simulink model "six_plus_six_AcmsteeringV10_main"  (R2014a)
settings: Solver=FixedStepDiscrete  StartTime=0.0  StopTime=10.0  FixedStep=0.0005  RelTol=1e-3
InitFcn:
  | Veh_Par_wxt
values from neighbouring files (symbols this model uses):
  acc_spdctl = [0 100]    [Veh_Par_wxt.m]
  ag_thr = ecucoder_cal(ag_thr)    [Veh_Par_wxt.m]
  B = 1.8    [Veh_Par_wxt.m]
  bra_em = 100    [Veh_Par_wxt.m]
  bra_pre_gz2 = 100/3    (= 33.3333333333)    [Veh_Par_wxt.m]
  bra_pre_gz34 = 10/3    (= 3.33333333333)    [Veh_Par_wxt.m]
  bra_pre_yd = 10/2    (= 5)    [Veh_Par_wxt.m]
  brakepre_dem_data = [0 1 2 3 4 5 6 7 8 9 10]    [Veh_Par_wxt.m]
  brakeTrq_dem_data = [0 125 251 376 502 627 753 878 1004 1129 1255]    [Veh_Par_wxt.m]
  bratrq_max = 4*1255    (= 5020)    [Veh_Par_wxt.m]
  eff_tran = 0.9    [Veh_Par_wxt.m]
  ESP_switch = ecucoder_cal(ESP_switch)    [Veh_Par_wxt.m]
  G = Mass*g    (= 15696)    [Veh_Par_wxt.m]
  kd1 = ecucoder_cal(kd1)    [Veh_Par_wxt.m]
  kd2 = 0    [Veh_Par_wxt.m]
  ki1 = ecucoder_cal(ki1)    [Veh_Par_wxt.m]
  ki2 = 1    [Veh_Par_wxt.m]
  kp1 = ecucoder_cal(kp1)    [Veh_Par_wxt.m]
  kp2 = 300    [Veh_Par_wxt.m]
  L = L1+L2    (= 2.9)    [Veh_Par_wxt.m]
  premax = 100    [Veh_Par_wxt.m]
  Radius = 0.4572/2    (= 0.2286)    [Veh_Par_wxt.m]
  RC_switch = ecucoder_cal(RC_switch)    [Veh_Par_wxt.m]
  s_opt_yi = 0.15    [Veh_Par_wxt.m]
  s_opt_zhuan = 0.8    [Veh_Par_wxt.m]
  s_opt_zhuan_add = 0.05    [Veh_Par_wxt.m]
  s_opt_zhuan_table = [0.8 0.8 0.3 0.3]    [Veh_Par_wxt.m]
  spd_map_mot = [0 499.85 999.79 1500 2000 2500 3000 3500 4000 4500 4999.8 5999.8]    [Veh_Par_wxt.m]
  spd_spdctl = [0 500]    [Veh_Par_wxt.m]
  speed_thr_park = 5/3.6/Radius*tras_ratio*30/pi    (= 464.143899364)    [Veh_Par_wxt.m]
  TCS_switch = ecucoder_cal(TCS_switch)    [Veh_Par_wxt.m]
  tras_ratio = 8    [Veh_Par_wxt.m]
  trq_map_mot = [70.5 70.012 71.154 65.797 53.917 45.159 38.073 32.685 27.48 17.133 14.949 10.07]    [Veh_Par_wxt.m]
  trqmax_yd = 70.5    [Veh_Par_wxt.m]
  trqmax_zx = 70.5    [Veh_Par_wxt.m]
  trqmaxneg = -70.5    [Veh_Par_wxt.m]
  v_gain = 0.9    [Veh_Par_wxt.m]
  v_table = [0 5 20 100]    [Veh_Par_wxt.m]
  v_thr_park = 5    [Veh_Par_wxt.m]
  zhidong_bianmazhi = [-140000 750000]    [Veh_Par_wxt.m]
  zhidong_down = -140000    [Veh_Par_wxt.m]
  zhidong_up = 750000    [Veh_Par_wxt.m]
  zhidong_youmen = [0 100]    [Veh_Par_wxt.m]
  zhuanxiang_bianmazhi = [-400000 0 400000]    [Veh_Par_wxt.m]
  zhuanxiang_down = -400000    [Veh_Par_wxt.m]
  zhuanxiang_up = 400000    [Veh_Par_wxt.m]
  zhuanxiang_youmen = [-100 0 100]    [Veh_Par_wxt.m]
undefined symbols (not defined in the file or in its folder): ecucoder_acal, guzhang_lf, guzhang_lm, guzhang_lr, guzhang_rf, guzhang_rm, guzhang_rr, myFIS
libraries: simulink x979, ec5744lib x59, fuzblock x2
(part 13 of 27)

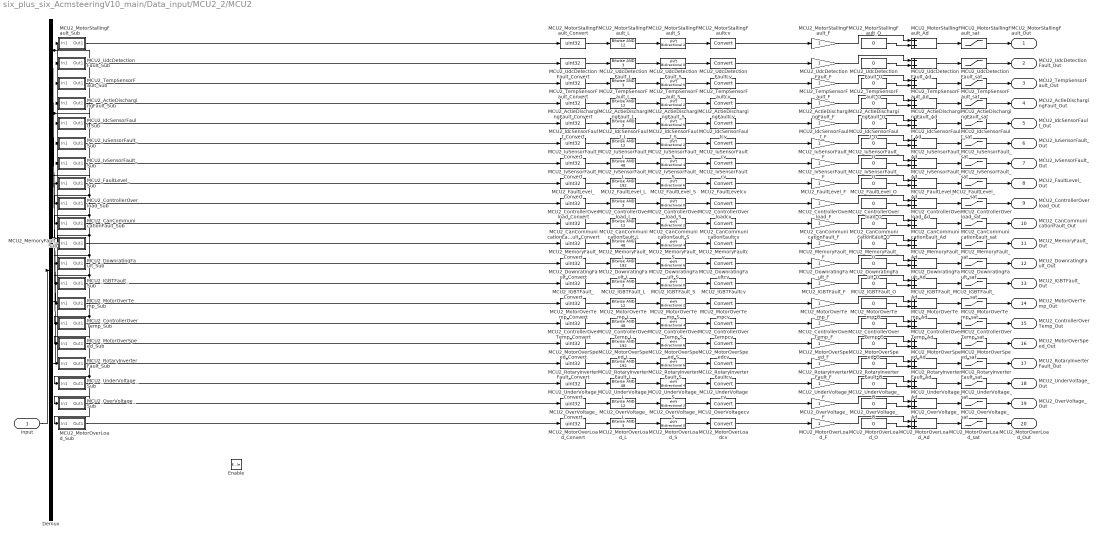
== system six_plus_six_AcmsteeringV10_main/Data_input/MCU2_2/MCU2 ==
  input : Inport
  Enable : EnablePort
  Demux : Demux  Outputs=8
  MCU2_ActieDischargingFault_Ad : Sum
  MCU2_ActieDischargingFault_Convert : DataTypeConversion  OutDataTypeStr=uint32
  MCU2_ActieDischargingFault_F : Gain
  MCU2_ActieDischargingFault_L : simulink/Logic and Bit Operations/Bitwise Operator  logicop=AND  UseBitMask=on  BitMask=12  BitMaskRealWorld=Stored Integer
  MCU2_ActieDischargingFault_O : Constant  Value=0  OutDataTypeStr=single
  MCU2_ActieDischargingFault_S : ArithShift  BitShiftNumber=2
  MCU2_ActieDischargingFault_Sub : Subsystem
  MCU2_ActieDischargingFault_sat : Saturate  UpperLimit=3  LowerLimit=0
  MCU2_ActieDischargingFaultcv : DataTypeConversion
  MCU2_CanCommunicationFault_Ad : Sum
  MCU2_CanCommunicationFault_Convert : DataTypeConversion  OutDataTypeStr=uint32
  MCU2_CanCommunicationFault_F : Gain
  MCU2_CanCommunicationFault_L : simulink/Logic and Bit Operations/Bitwise Operator  logicop=AND  UseBitMask=on  BitMask=12  BitMaskRealWorld=Stored Integer
  MCU2_CanCommunicationFault_O : Constant  Value=0  OutDataTypeStr=single
  MCU2_CanCommunicationFault_S : ArithShift  BitShiftNumber=2
  MCU2_CanCommunicationFault_Sub : Subsystem
  MCU2_CanCommunicationFault_sat : Saturate  UpperLimit=3  LowerLimit=0
  MCU2_CanCommunicationFaultcv : DataTypeConversion
  MCU2_ControllerOverTemp_Ad : Sum
  MCU2_ControllerOverTemp_Convert : DataTypeConversion  OutDataTypeStr=uint32
  MCU2_ControllerOverTemp_F : Gain
  MCU2_ControllerOverTemp_L : simulink/Logic and Bit Operations/Bitwise Operator  logicop=AND  UseBitMask=on  BitMask=48  BitMaskRealWorld=Stored Integer
  MCU2_ControllerOverTemp_O : Constant  Value=0  OutDataTypeStr=single
  MCU2_ControllerOverTemp_S : ArithShift  BitShiftNumber=4
  MCU2_ControllerOverTemp_Sub : Subsystem
  MCU2_ControllerOverTemp_sat : Saturate  UpperLimit=3  LowerLimit=0
  MCU2_ControllerOverTempcv : DataTypeConversion
  MCU2_ControllerOverload_Ad : Sum
  MCU2_ControllerOverload_Convert : DataTypeConversion  OutDataTypeStr=uint32
  MCU2_ControllerOverload_F : Gain
  MCU2_ControllerOverload_L : simulink/Logic and Bit Operations/Bitwise Operator  logicop=AND  UseBitMask=on  BitMask=3  BitMaskRealWorld=Stored Integer
  MCU2_ControllerOverload_O : Constant  Value=0  OutDataTypeStr=single
  MCU2_ControllerOverload_S : ArithShift
  MCU2_ControllerOverload_Sub : Subsystem
  MCU2_ControllerOverload_sat : Saturate  UpperLimit=3  LowerLimit=0
  MCU2_ControllerOverloadcv : DataTypeConversion
  MCU2_DownratingFault_Ad : Sum
  MCU2_DownratingFault_Convert : DataTypeConversion  OutDataTypeStr=uint32
  MCU2_DownratingFault_F : Gain
  MCU2_DownratingFault_L : simulink/Logic and Bit Operations/Bitwise Operator  logicop=AND  UseBitMask=on  BitMask=192  BitMaskRealWorld=Stored Integer
  MCU2_DownratingFault_O : Constant  Value=0  OutDataTypeStr=single
  MCU2_DownratingFault_S : ArithShift  BitShiftNumber=6
  MCU2_DownratingFault_Sub : Subsystem
  MCU2_DownratingFault_sat : Saturate  UpperLimit=3  LowerLimit=0
  MCU2_DownratingFaultcv : DataTypeConversion
  MCU2_FaultLevel_Ad : Sum
  MCU2_FaultLevel_Convert : DataTypeConversion  OutDataTypeStr=uint32
  MCU2_FaultLevel_F : Gain
  MCU2_FaultLevel_L : simulink/Logic and Bit Operations/Bitwise Operator  logicop=AND  UseBitMask=on  BitMask=192  BitMaskRealWorld=Stored Integer
  MCU2_FaultLevel_O : Constant  Value=0  OutDataTypeStr=single
  MCU2_FaultLevel_S : ArithShift  BitShiftNumber=6
  MCU2_FaultLevel_Sub : Subsystem
  MCU2_FaultLevel_sat : Saturate  UpperLimit=3  LowerLimit=0
  MCU2_FaultLevelcv : DataTypeConversion
  MCU2_IGBTFault_Ad : Sum
  MCU2_IGBTFault_Convert : DataTypeConversion  OutDataTypeStr=uint32
  MCU2_IGBTFault_F : Gain
  MCU2_IGBTFault_L : simulink/Logic and Bit Operations/Bitwise Operator  logicop=AND  UseBitMask=on  BitMask=3  BitMaskRealWorld=Stored Integer
  MCU2_IGBTFault_O : Constant  Value=0  OutDataTypeStr=single
  MCU2_IGBTFault_S : ArithShift
  MCU2_IGBTFault_Sub : Subsystem
  MCU2_IGBTFault_sat : Saturate  UpperLimit=3  LowerLimit=0
  MCU2_IGBTFaultcv : DataTypeConversion
  MCU2_IdcSensorFault_Ad : Sum
  MCU2_IdcSensorFault_Convert : DataTypeConversion  OutDataTypeStr=uint32
  MCU2_IdcSensorFault_F : Gain
  MCU2_IdcSensorFault_L : simulink/Logic and Bit Operations/Bitwise Operator  logicop=AND  UseBitMask=on  BitMask=3  BitMaskRealWorld=Stored Integer
  MCU2_IdcSensorFault_O : Constant  Value=0  OutDataTypeStr=single
  MCU2_IdcSensorFault_S : ArithShift
  MCU2_IdcSensorFault_Sub : Subsystem
  MCU2_IdcSensorFault_sat : Saturate  UpperLimit=3  LowerLimit=0
  MCU2_IdcSensorFaultcv : DataTypeConversion
  MCU2_IuSensorFault_Ad : Sum
  MCU2_IuSensorFault_Convert : DataTypeConversion  OutDataTypeStr=uint32
  MCU2_IuSensorFault_F : Gain
  MCU2_IuSensorFault_L : simulink/Logic and Bit Operations/Bitwise Operator  logicop=AND  UseBitMask=on  BitMask=12  BitMaskRealWorld=Stored Integer
  MCU2_IuSensorFault_O : Constant  Value=0  OutDataTypeStr=single
  MCU2_IuSensorFault_S : ArithShift  BitShiftNumber=2
  MCU2_IuSensorFault_Sub : Subsystem
  MCU2_IuSensorFault_sat : Saturate  UpperLimit=3  LowerLimit=0
  MCU2_IuSensorFaultcv : DataTypeConversion
  MCU2_IvSensorFault_Ad : Sum
  MCU2_IvSensorFault_Convert : DataTypeConversion  OutDataTypeStr=uint32
  MCU2_IvSensorFault_F : Gain
  MCU2_IvSensorFault_L : simulink/Logic and Bit Operations/Bitwise Operator  logicop=AND  UseBitMask=on  BitMask=48  BitMaskRealWorld=Stored Integer
  MCU2_IvSensorFault_O : Constant  Value=0  OutDataTypeStr=single
  MCU2_IvSensorFault_S : ArithShift  BitShiftNumber=4
  MCU2_IvSensorFault_Sub : Subsystem
  MCU2_IvSensorFault_sat : Saturate  UpperLimit=3  LowerLimit=0
  MCU2_IvSensorFaultcv : DataTypeConversion
  MCU2_MemoryFault_Ad : Sum
  MCU2_MemoryFault_Convert : DataTypeConversion  OutDataTypeStr=uint32
  MCU2_MemoryFault_F : Gain
  MCU2_MemoryFault_L : simulink/Logic and Bit Operations/Bitwise Operator  logicop=AND  UseBitMask=on  BitMask=48  BitMaskRealWorld=Stored Integer
  MCU2_MemoryFault_O : Constant  Value=0  OutDataTypeStr=single
  MCU2_MemoryFault_S : ArithShift  BitShiftNumber=4
  MCU2_MemoryFault_Sub : Subsystem
  MCU2_MemoryFault_sat : Saturate  UpperLimit=3  LowerLimit=0
  MCU2_MemoryFaultcv : DataTypeConversion
  MCU2_MotorOverLoad_Ad : Sum
  MCU2_MotorOverLoad_Convert : DataTypeConversion  OutDataTypeStr=uint32
  MCU2_MotorOverLoad_F : Gain
  MCU2_MotorOverLoad_L : simulink/Logic and Bit Operations/Bitwise Operator  logicop=AND  UseBitMask=on  BitMask=3  BitMaskRealWorld=Stored Integer
  MCU2_MotorOverLoad_O : Constant  Value=0  OutDataTypeStr=single
  MCU2_MotorOverLoad_S : ArithShift
  MCU2_MotorOverLoad_Sub : Subsystem
  MCU2_MotorOverLoad_sat : Saturate  UpperLimit=3  LowerLimit=0
  MCU2_MotorOverLoadcv : DataTypeConversion
  MCU2_MotorOverSpeed_Ad : Sum
  MCU2_MotorOverSpeed_Convert : DataTypeConversion  OutDataTypeStr=uint32
  MCU2_MotorOverSpeed_F : Gain
  MCU2_MotorOverSpeed_L : simulink/Logic and Bit Operations/Bitwise Operator  logicop=AND  UseBitMask=on  BitMask=192  BitMaskRealWorld=Stored Integer
  MCU2_MotorOverSpeed_O : Constant  Value=0  OutDataTypeStr=single
  MCU2_MotorOverSpeed_S : ArithShift  BitShiftNumber=6
  MCU2_MotorOverSpeed_Sub : Subsystem
  MCU2_MotorOverSpeed_sat : Saturate  UpperLimit=3  LowerLimit=0
  MCU2_MotorOverSpeedcv : DataTypeConversion
  MCU2_MotorOverTemp_Ad : Sum
  MCU2_MotorOverTemp_Convert : DataTypeConversion  OutDataTypeStr=uint32
  MCU2_MotorOverTemp_F : Gain
  MCU2_MotorOverTemp_L : simulink/Logic and Bit Operations/Bitwise Operator  logicop=AND  UseBitMask=on  BitMask=12  BitMaskRealWorld=Stored Integer
  MCU2_MotorOverTemp_O : Constant  Value=0  OutDataTypeStr=single
  MCU2_MotorOverTemp_S : ArithShift  BitShiftNumber=2
  MCU2_MotorOverTemp_Sub : Subsystem
  MCU2_MotorOverTemp_sat : Saturate  UpperLimit=3  LowerLimit=0
  MCU2_MotorOverTempcv : DataTypeConversion
  MCU2_MotorStallingFault_Ad : Sum
  MCU2_MotorStallingFault_Convert : DataTypeConversion  OutDataTypeStr=uint32
  MCU2_MotorStallingFault_F : Gain
  MCU2_MotorStallingFault_L : simulink/Logic and Bit Operations/Bitwise Operator  logicop=AND  UseBitMask=on  BitMask=12  BitMaskRealWorld=Stored Integer
  MCU2_MotorStallingFault_O : Constant  Value=0  OutDataTypeStr=single
  MCU2_MotorStallingFault_S : ArithShift  BitShiftNumber=2
  MCU2_MotorStallingFault_Sub : Subsystem
  MCU2_MotorStallingFault_sat : Saturate  UpperLimit=3  LowerLimit=0
  MCU2_MotorStallingFaultcv : DataTypeConversion
  MCU2_OverVoltage_Ad : Sum
  MCU2_OverVoltage_Convert : DataTypeConversion  OutDataTypeStr=uint32
  MCU2_OverVoltage_F : Gain
  MCU2_OverVoltage_L : simulink/Logic and Bit Operations/Bitwise Operator  logicop=AND  UseBitMask=on  BitMask=12  BitMaskRealWorld=Stored Integer
  MCU2_OverVoltage_O : Constant  Value=0  OutDataTypeStr=single
  MCU2_OverVoltage_S : ArithShift  BitShiftNumber=2
  MCU2_OverVoltage_Sub : Subsystem
  MCU2_OverVoltage_sat : Saturate  UpperLimit=3  LowerLimit=0
  MCU2_OverVoltagecv : DataTypeConversion
  MCU2_RotaryInverterFault_Ad : Sum
  MCU2_RotaryInverterFault_Convert : DataTypeConversion  OutDataTypeStr=uint32
  MCU2_RotaryInverterFault_F : Gain
  MCU2_RotaryInverterFault_L : simulink/Logic and Bit Operations/Bitwise Operator  logicop=AND  UseBitMask=on  BitMask=192  BitMaskRealWorld=Stored Integer
  MCU2_RotaryInverterFault_O : Constant  Value=0  OutDataTypeStr=single
  MCU2_RotaryInverterFault_S : ArithShift  BitShiftNumber=6
  MCU2_RotaryInverterFault_Sub : Subsystem
  MCU2_RotaryInverterFault_sat : Saturate  UpperLimit=3  LowerLimit=0
  MCU2_RotaryInverterFaultcv : DataTypeConversion
  MCU2_TempSensorFault_Ad : Sum
  MCU2_TempSensorFault_Convert : DataTypeConversion  OutDataTypeStr=uint32
  MCU2_TempSensorFault_F : Gain
  MCU2_TempSensorFault_L : simulink/Logic and Bit Operations/Bitwise Operator  logicop=AND  UseBitMask=on  BitMask=3  BitMaskRealWorld=Stored Integer
  MCU2_TempSensorFault_O : Constant  Value=0  OutDataTypeStr=single
  MCU2_TempSensorFault_S : ArithShift
  MCU2_TempSensorFault_Sub : Subsystem
  MCU2_TempSensorFault_sat : Saturate  UpperLimit=3  LowerLimit=0
  MCU2_TempSensorFaultcv : DataTypeConversion
  MCU2_UdcDetectionFault_Ad : Sum
  MCU2_UdcDetectionFault_Convert : DataTypeConversion  OutDataTypeStr=uint32
  MCU2_UdcDetectionFault_F : Gain
  MCU2_UdcDetectionFault_L : simulink/Logic and Bit Operations/Bitwise Operator  logicop=AND  UseBitMask=on  BitMask=3  BitMaskRealWorld=Stored Integer
  MCU2_UdcDetectionFault_O : Constant  Value=0  OutDataTypeStr=single
  MCU2_UdcDetectionFault_S : ArithShift
  MCU2_UdcDetectionFault_Sub : Subsystem
  MCU2_UdcDetectionFault_sat : Saturate  UpperLimit=3  LowerLimit=0
  MCU2_UdcDetectionFaultcv : DataTypeConversion
  MCU2_UnderVoltage_Ad : Sum
  MCU2_UnderVoltage_Convert : DataTypeConversion  OutDataTypeStr=uint32
  MCU2_UnderVoltage_F : Gain
  MCU2_UnderVoltage_L : simulink/Logic and Bit Operations/Bitwise Operator  logicop=AND  UseBitMask=on  BitMask=48  BitMaskRealWorld=Stored Integer
  MCU2_UnderVoltage_O : Constant  Value=0  OutDataTypeStr=single
  MCU2_UnderVoltage_S : ArithShift  BitShiftNumber=4
  MCU2_UnderVoltage_Sub : Subsystem
  MCU2_UnderVoltage_sat : Saturate  UpperLimit=3  LowerLimit=0
  MCU2_UnderVoltagecv : DataTypeConversion
  MCU2_MotorStallingFault_Out : Outport
  MCU2_UdcDetectionFault_Out : Outport  Port=2
  MCU2_TempSensorFault_Out : Outport  Port=3
  MCU2_ActieDischargingFault_Out : Outport  Port=4
  MCU2_IdcSensorFault_Out : Outport  Port=5
  MCU2_IuSensorFault_Out : Outport  Port=6
  MCU2_IvSensorFault_Out : Outport  Port=7
  MCU2_FaultLevel_Out : Outport  Port=8
  MCU2_ControllerOverload_Out : Outport  Port=9
  MCU2_CanCommunicationFault_Out : Outport  Port=10
  MCU2_MemoryFault_Out : Outport  Port=11
  MCU2_DownratingFault_Out : Outport  Port=12
  MCU2_IGBTFault_Out : Outport  Port=13
  MCU2_MotorOverTemp_Out : Outport  Port=14
  MCU2_ControllerOverTemp_Out : Outport  Port=15
  MCU2_MotorOverSpeed_Out : Outport  Port=16
  MCU2_RotaryInverterFault_Out : Outport  Port=17
  MCU2_UnderVoltage_Out : Outport  Port=18
  MCU2_OverVoltage_Out : Outport  Port=19
  MCU2_MotorOverLoad_Out : Outport  Port=20
  wires:
  MCU2_MotorStallingFault_F/1 -> MCU2_MotorStallingFault_Ad/1
  MCU2_MotorStallingFault_O/1 -> MCU2_MotorStallingFault_Ad/2
  MCU2_MotorStallingFault_Ad/1 -> MCU2_MotorStallingFault_sat/1
  MCU2_MotorStallingFault_sat/1 -> MCU2_MotorStallingFault_Out/1
  Demux/6 -> MCU2_MotorStallingFault_Sub/1(In1), MCU2_UdcDetectionFault_Sub/1(In1)
  MCU2_MotorStallingFault_Sub/1(Out1) -> MCU2_MotorStallingFault_Convert/1
  MCU2_MotorStallingFault_Convert/1 -> MCU2_MotorStallingFault_L/1
  MCU2_MotorStallingFault_L/1 -> MCU2_MotorStallingFault_S/1
  MCU2_MotorStallingFault_S/1 -> MCU2_MotorStallingFaultcv/1
  MCU2_MotorStallingFaultcv/1 -> MCU2_MotorStallingFault_F/1
  MCU2_UdcDetectionFault_F/1 -> MCU2_UdcDetectionFault_Ad/1
  MCU2_UdcDetectionFault_O/1 -> MCU2_UdcDetectionFault_Ad/2
  MCU2_UdcDetectionFault_Ad/1 -> MCU2_UdcDetectionFault_sat/1
  MCU2_UdcDetectionFault_sat/1 -> MCU2_UdcDetectionFault_Out/1
  MCU2_UdcDetectionFault_Sub/1(Out1) -> MCU2_UdcDetectionFault_Convert/1
  MCU2_UdcDetectionFault_Convert/1 -> MCU2_UdcDetectionFault_L/1
  MCU2_UdcDetectionFault_L/1 -> MCU2_UdcDetectionFault_S/1
  MCU2_UdcDetectionFault_S/1 -> MCU2_UdcDetectionFaultcv/1
  MCU2_UdcDetectionFaultcv/1 -> MCU2_UdcDetectionFault_F/1
  MCU2_TempSensorFault_F/1 -> MCU2_TempSensorFault_Ad/1
  MCU2_TempSensorFault_O/1 -> MCU2_TempSensorFault_Ad/2
  MCU2_TempSensorFault_Ad/1 -> MCU2_TempSensorFault_sat/1
  MCU2_TempSensorFault_sat/1 -> MCU2_TempSensorFault_Out/1
  Demux/5 -> MCU2_TempSensorFault_Sub/1(In1), MCU2_ActieDischargingFault_Sub/1(In1)
  MCU2_TempSensorFault_Sub/1(Out1) -> MCU2_TempSensorFault_Convert/1
  MCU2_TempSensorFault_Convert/1 -> MCU2_TempSensorFault_L/1
  MCU2_TempSensorFault_L/1 -> MCU2_TempSensorFault_S/1
  MCU2_TempSensorFault_S/1 -> MCU2_TempSensorFaultcv/1
  MCU2_TempSensorFaultcv/1 -> MCU2_TempSensorFault_F/1
  MCU2_ActieDischargingFault_F/1 -> MCU2_ActieDischargingFault_Ad/1
  MCU2_ActieDischargingFault_O/1 -> MCU2_ActieDischargingFault_Ad/2
  MCU2_ActieDischargingFault_Ad/1 -> MCU2_ActieDischargingFault_sat/1
  MCU2_ActieDischargingFault_sat/1 -> MCU2_ActieDischargingFault_Out/1
  MCU2_ActieDischargingFault_Sub/1(Out1) -> MCU2_ActieDischargingFault_Convert/1
  MCU2_ActieDischargingFault_Convert/1 -> MCU2_ActieDischargingFault_L/1
  MCU2_ActieDischargingFault_L/1 -> MCU2_ActieDischargingFault_S/1
  MCU2_ActieDischargingFault_S/1 -> MCU2_ActieDischargingFaultcv/1
  MCU2_ActieDischargingFaultcv/1 -> MCU2_ActieDischargingFault_F/1
  MCU2_IdcSensorFault_F/1 -> MCU2_IdcSensorFault_Ad/1
  MCU2_IdcSensorFault_O/1 -> MCU2_IdcSensorFault_Ad/2
  MCU2_IdcSensorFault_Ad/1 -> MCU2_IdcSensorFault_sat/1
  MCU2_IdcSensorFault_sat/1 -> MCU2_IdcSensorFault_Out/1
  Demux/4 -> MCU2_IdcSensorFault_Sub/1(In1), MCU2_IuSensorFault_Sub/1(In1), MCU2_IvSensorFault_Sub/1(In1), MCU2_FaultLevel_Sub/1(In1)
  MCU2_IdcSensorFault_Sub/1(Out1) -> MCU2_IdcSensorFault_Convert/1
  MCU2_IdcSensorFault_Convert/1 -> MCU2_IdcSensorFault_L/1
  MCU2_IdcSensorFault_L/1 -> MCU2_IdcSensorFault_S/1
  MCU2_IdcSensorFault_S/1 -> MCU2_IdcSensorFaultcv/1
  MCU2_IdcSensorFaultcv/1 -> MCU2_IdcSensorFault_F/1
  MCU2_IuSensorFault_F/1 -> MCU2_IuSensorFault_Ad/1
  MCU2_IuSensorFault_O/1 -> MCU2_IuSensorFault_Ad/2
  MCU2_IuSensorFault_Ad/1 -> MCU2_IuSensorFault_sat/1
  MCU2_IuSensorFault_sat/1 -> MCU2_IuSensorFault_Out/1
  MCU2_IuSensorFault_Sub/1(Out1) -> MCU2_IuSensorFault_Convert/1
  MCU2_IuSensorFault_Convert/1 -> MCU2_IuSensorFault_L/1
  MCU2_IuSensorFault_L/1 -> MCU2_IuSensorFault_S/1
  MCU2_IuSensorFault_S/1 -> MCU2_IuSensorFaultcv/1
  MCU2_IuSensorFaultcv/1 -> MCU2_IuSensorFault_F/1
  MCU2_IvSensorFault_F/1 -> MCU2_IvSensorFault_Ad/1
  MCU2_IvSensorFault_O/1 -> MCU2_IvSensorFault_Ad/2
  MCU2_IvSensorFault_Ad/1 -> MCU2_IvSensorFault_sat/1
  MCU2_IvSensorFault_sat/1 -> MCU2_IvSensorFault_Out/1
  MCU2_IvSensorFault_Sub/1(Out1) -> MCU2_IvSensorFault_Convert/1
  MCU2_IvSensorFault_Convert/1 -> MCU2_IvSensorFault_L/1
  MCU2_IvSensorFault_L/1 -> MCU2_IvSensorFault_S/1
  MCU2_IvSensorFault_S/1 -> MCU2_IvSensorFaultcv/1
  MCU2_IvSensorFaultcv/1 -> MCU2_IvSensorFault_F/1
  MCU2_FaultLevel_F/1 -> MCU2_FaultLevel_Ad/1
  MCU2_FaultLevel_O/1 -> MCU2_FaultLevel_Ad/2
  MCU2_FaultLevel_Ad/1 -> MCU2_FaultLevel_sat/1
  MCU2_FaultLevel_sat/1 -> MCU2_FaultLevel_Out/1
  MCU2_FaultLevel_Sub/1(Out1) -> MCU2_FaultLevel_Convert/1
  MCU2_FaultLevel_Convert/1 -> MCU2_FaultLevel_L/1
  MCU2_FaultLevel_L/1 -> MCU2_FaultLevel_S/1
  MCU2_FaultLevel_S/1 -> MCU2_FaultLevelcv/1
  MCU2_FaultLevelcv/1 -> MCU2_FaultLevel_F/1
  MCU2_ControllerOverload_F/1 -> MCU2_ControllerOverload_Ad/1
  MCU2_ControllerOverload_O/1 -> MCU2_ControllerOverload_Ad/2
  MCU2_ControllerOverload_Ad/1 -> MCU2_ControllerOverload_sat/1
  MCU2_ControllerOverload_sat/1 -> MCU2_ControllerOverload_Out/1
  Demux/1 -> MCU2_UnderVoltage_Sub/1(In1), MCU2_OverVoltage_Sub/1(In1), MCU2_ControllerOverload_Sub/1(In1), MCU2_RotaryInverterFault_Sub/1(In1)
  MCU2_ControllerOverload_Sub/1(Out1) -> MCU2_ControllerOverload_Convert/1
  MCU2_ControllerOverload_Convert/1 -> MCU2_ControllerOverload_L/1
  MCU2_ControllerOverload_L/1 -> MCU2_ControllerOverload_S/1
  MCU2_ControllerOverload_S/1 -> MCU2_ControllerOverloadcv/1
  MCU2_ControllerOverloadcv/1 -> MCU2_ControllerOverload_F/1
  MCU2_CanCommunicationFault_F/1 -> MCU2_CanCommunicationFault_Ad/1
  MCU2_CanCommunicationFault_O/1 -> MCU2_CanCommunicationFault_Ad/2
  MCU2_CanCommunicationFault_Ad/1 -> MCU2_CanCommunicationFault_sat/1
  MCU2_CanCommunicationFault_sat/1 -> MCU2_CanCommunicationFault_Out/1
  Demux/3 -> MCU2_DownratingFault_Sub/1(In1), MCU2_MotorOverLoad_Sub/1(In1), MCU2_MemoryFault_Sub/1(In1), MCU2_CanCommunicationFault_Sub/1(In1)
  MCU2_CanCommunicationFault_Sub/1(Out1) -> MCU2_CanCommunicationFault_Convert/1
  MCU2_CanCommunicationFault_Convert/1 -> MCU2_CanCommunicationFault_L/1
  MCU2_CanCommunicationFault_L/1 -> MCU2_CanCommunicationFault_S/1
  MCU2_CanCommunicationFault_S/1 -> MCU2_CanCommunicationFaultcv/1
  MCU2_CanCommunicationFaultcv/1 -> MCU2_CanCommunicationFault_F/1
  MCU2_MemoryFault_F/1 -> MCU2_MemoryFault_Ad/1
  MCU2_MemoryFault_O/1 -> MCU2_MemoryFault_Ad/2
  MCU2_MemoryFault_Ad/1 -> MCU2_MemoryFault_sat/1
  MCU2_MemoryFault_sat/1 -> MCU2_MemoryFault_Out/1
  MCU2_MemoryFault_Sub/1(Out1) -> MCU2_MemoryFault_Convert/1
  MCU2_MemoryFault_Convert/1 -> MCU2_MemoryFault_L/1
  MCU2_MemoryFault_L/1 -> MCU2_MemoryFault_S/1
  MCU2_MemoryFault_S/1 -> MCU2_MemoryFaultcv/1
  MCU2_MemoryFaultcv/1 -> MCU2_MemoryFault_F/1
  MCU2_DownratingFault_F/1 -> MCU2_DownratingFault_Ad/1
  MCU2_DownratingFault_O/1 -> MCU2_DownratingFault_Ad/2
  MCU2_DownratingFault_Ad/1 -> MCU2_DownratingFault_sat/1
  MCU2_DownratingFault_sat/1 -> MCU2_DownratingFault_Out/1
  MCU2_DownratingFault_Sub/1(Out1) -> MCU2_DownratingFault_Convert/1
  MCU2_DownratingFault_Convert/1 -> MCU2_DownratingFault_L/1
  MCU2_DownratingFault_L/1 -> MCU2_DownratingFault_S/1
  MCU2_DownratingFault_S/1 -> MCU2_DownratingFaultcv/1
  MCU2_DownratingFaultcv/1 -> MCU2_DownratingFault_F/1
  MCU2_IGBTFault_F/1 -> MCU2_IGBTFault_Ad/1
  MCU2_IGBTFault_O/1 -> MCU2_IGBTFault_Ad/2
  MCU2_IGBTFault_Ad/1 -> MCU2_IGBTFault_sat/1
  MCU2_IGBTFault_sat/1 -> MCU2_IGBTFault_Out/1
  Demux/2 -> MCU2_ControllerOverTemp_Sub/1(In1), MCU2_MotorOverSpeed_Sub/1(In1), MCU2_IGBTFault_Sub/1(In1), MCU2_MotorOverTemp_Sub/1(In1)
  MCU2_IGBTFault_Sub/1(Out1) -> MCU2_IGBTFault_Convert/1
  MCU2_IGBTFault_Convert/1 -> MCU2_IGBTFault_L/1
  MCU2_IGBTFault_L/1 -> MCU2_IGBTFault_S/1
  MCU2_IGBTFault_S/1 -> MCU2_IGBTFaultcv/1
  MCU2_IGBTFaultcv/1 -> MCU2_IGBTFault_F/1
  MCU2_MotorOverTemp_F/1 -> MCU2_MotorOverTemp_Ad/1
  MCU2_MotorOverTemp_O/1 -> MCU2_MotorOverTemp_Ad/2
  MCU2_MotorOverTemp_Ad/1 -> MCU2_MotorOverTemp_sat/1
  MCU2_MotorOverTemp_sat/1 -> MCU2_MotorOverTemp_Out/1
  MCU2_MotorOverTemp_Sub/1(Out1) -> MCU2_MotorOverTemp_Convert/1
  MCU2_MotorOverTemp_Convert/1 -> MCU2_MotorOverTemp_L/1
  MCU2_MotorOverTemp_L/1 -> MCU2_MotorOverTemp_S/1
  MCU2_MotorOverTemp_S/1 -> MCU2_MotorOverTempcv/1
  MCU2_MotorOverTempcv/1 -> MCU2_MotorOverTemp_F/1
  MCU2_ControllerOverTemp_F/1 -> MCU2_ControllerOverTemp_Ad/1
  MCU2_ControllerOverTemp_O/1 -> MCU2_ControllerOverTemp_Ad/2
  MCU2_ControllerOverTemp_Ad/1 -> MCU2_ControllerOverTemp_sat/1
  MCU2_ControllerOverTemp_sat/1 -> MCU2_ControllerOverTemp_Out/1
  MCU2_ControllerOverTemp_Sub/1(Out1) -> MCU2_ControllerOverTemp_Convert/1
  MCU2_ControllerOverTemp_Convert/1 -> MCU2_ControllerOverTemp_L/1
  MCU2_ControllerOverTemp_L/1 -> MCU2_ControllerOverTemp_S/1
  MCU2_ControllerOverTemp_S/1 -> MCU2_ControllerOverTempcv/1
  MCU2_ControllerOverTempcv/1 -> MCU2_ControllerOverTemp_F/1
  MCU2_MotorOverSpeed_F/1 -> MCU2_MotorOverSpeed_Ad/1
  MCU2_MotorOverSpeed_O/1 -> MCU2_MotorOverSpeed_Ad/2
  MCU2_MotorOverSpeed_Ad/1 -> MCU2_MotorOverSpeed_sat/1
  MCU2_MotorOverSpeed_sat/1 -> MCU2_MotorOverSpeed_Out/1
  MCU2_MotorOverSpeed_Sub/1(Out1) -> MCU2_MotorOverSpeed_Convert/1
  MCU2_MotorOverSpeed_Convert/1 -> MCU2_MotorOverSpeed_L/1
  MCU2_MotorOverSpeed_L/1 -> MCU2_MotorOverSpeed_S/1
  MCU2_MotorOverSpeed_S/1 -> MCU2_MotorOverSpeedcv/1
  MCU2_MotorOverSpeedcv/1 -> MCU2_MotorOverSpeed_F/1
  MCU2_RotaryInverterFault_F/1 -> MCU2_RotaryInverterFault_Ad/1
  MCU2_RotaryInverterFault_O/1 -> MCU2_RotaryInverterFault_Ad/2
  MCU2_RotaryInverterFault_Ad/1 -> MCU2_RotaryInverterFault_sat/1
  MCU2_RotaryInverterFault_sat/1 -> MCU2_RotaryInverterFault_Out/1
  MCU2_RotaryInverterFault_Sub/1(Out1) -> MCU2_RotaryInverterFault_Convert/1
  MCU2_RotaryInverterFault_Convert/1 -> MCU2_RotaryInverterFault_L/1
  MCU2_RotaryInverterFault_L/1 -> MCU2_RotaryInverterFault_S/1
  MCU2_RotaryInverterFault_S/1 -> MCU2_RotaryInverterFaultcv/1
  MCU2_RotaryInverterFaultcv/1 -> MCU2_RotaryInverterFault_F/1
  MCU2_UnderVoltage_F/1 -> MCU2_UnderVoltage_Ad/1
  MCU2_UnderVoltage_O/1 -> MCU2_UnderVoltage_Ad/2
  MCU2_UnderVoltage_Ad/1 -> MCU2_UnderVoltage_sat/1
  MCU2_UnderVoltage_sat/1 -> MCU2_UnderVoltage_Out/1
  MCU2_UnderVoltage_Sub/1(Out1) -> MCU2_UnderVoltage_Convert/1
  MCU2_UnderVoltage_Convert/1 -> MCU2_UnderVoltage_L/1
  MCU2_UnderVoltage_L/1 -> MCU2_UnderVoltage_S/1
  MCU2_UnderVoltage_S/1 -> MCU2_UnderVoltagecv/1
  MCU2_UnderVoltagecv/1 -> MCU2_UnderVoltage_F/1
  MCU2_OverVoltage_F/1 -> MCU2_OverVoltage_Ad/1
  MCU2_OverVoltage_O/1 -> MCU2_OverVoltage_Ad/2
  MCU2_OverVoltage_Ad/1 -> MCU2_OverVoltage_sat/1
  MCU2_OverVoltage_sat/1 -> MCU2_OverVoltage_Out/1
  MCU2_OverVoltage_Sub/1(Out1) -> MCU2_OverVoltage_Convert/1
  MCU2_OverVoltage_Convert/1 -> MCU2_OverVoltage_L/1
  MCU2_OverVoltage_L/1 -> MCU2_OverVoltage_S/1
  MCU2_OverVoltage_S/1 -> MCU2_OverVoltagecv/1
  MCU2_OverVoltagecv/1 -> MCU2_OverVoltage_F/1
  MCU2_MotorOverLoad_F/1 -> MCU2_MotorOverLoad_Ad/1
  MCU2_MotorOverLoad_O/1 -> MCU2_MotorOverLoad_Ad/2
  MCU2_MotorOverLoad_Ad/1 -> MCU2_MotorOverLoad_sat/1
  MCU2_MotorOverLoad_sat/1 -> MCU2_MotorOverLoad_Out/1
  MCU2_MotorOverLoad_Sub/1(Out1) -> MCU2_MotorOverLoad_Convert/1
  MCU2_MotorOverLoad_Convert/1 -> MCU2_MotorOverLoad_L/1
  MCU2_MotorOverLoad_L/1 -> MCU2_MotorOverLoad_S/1
  MCU2_MotorOverLoad_S/1 -> MCU2_MotorOverLoadcv/1
  MCU2_MotorOverLoadcv/1 -> MCU2_MotorOverLoad_F/1
  input/1 -> Demux/1

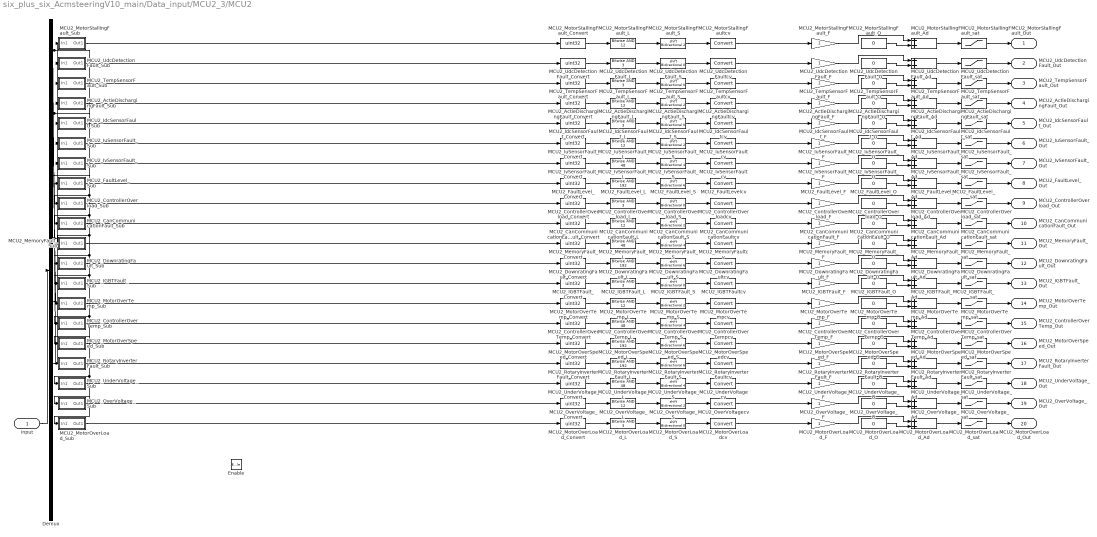
== system six_plus_six_AcmsteeringV10_main/Data_input/MCU2_3/MCU2 ==
  input : Inport
  Enable : EnablePort
  Demux : Demux  Outputs=8
  MCU2_ActieDischargingFault_Ad : Sum
  MCU2_ActieDischargingFault_Convert : DataTypeConversion  OutDataTypeStr=uint32
  MCU2_ActieDischargingFault_F : Gain
  MCU2_ActieDischargingFault_L : simulink/Logic and Bit Operations/Bitwise Operator  logicop=AND  UseBitMask=on  BitMask=12  BitMaskRealWorld=Stored Integer
  MCU2_ActieDischargingFault_O : Constant  Value=0  OutDataTypeStr=single
  MCU2_ActieDischargingFault_S : ArithShift  BitShiftNumber=2
  MCU2_ActieDischargingFault_Sub : Subsystem
  MCU2_ActieDischargingFault_sat : Saturate  UpperLimit=3  LowerLimit=0
  MCU2_ActieDischargingFaultcv : DataTypeConversion
  MCU2_CanCommunicationFault_Ad : Sum
  MCU2_CanCommunicationFault_Convert : DataTypeConversion  OutDataTypeStr=uint32
  MCU2_CanCommunicationFault_F : Gain
  MCU2_CanCommunicationFault_L : simulink/Logic and Bit Operations/Bitwise Operator  logicop=AND  UseBitMask=on  BitMask=12  BitMaskRealWorld=Stored Integer
  MCU2_CanCommunicationFault_O : Constant  Value=0  OutDataTypeStr=single
  MCU2_CanCommunicationFault_S : ArithShift  BitShiftNumber=2
  MCU2_CanCommunicationFault_Sub : Subsystem
  MCU2_CanCommunicationFault_sat : Saturate  UpperLimit=3  LowerLimit=0
  MCU2_CanCommunicationFaultcv : DataTypeConversion
  MCU2_ControllerOverTemp_Ad : Sum
  MCU2_ControllerOverTemp_Convert : DataTypeConversion  OutDataTypeStr=uint32
  MCU2_ControllerOverTemp_F : Gain
  MCU2_ControllerOverTemp_L : simulink/Logic and Bit Operations/Bitwise Operator  logicop=AND  UseBitMask=on  BitMask=48  BitMaskRealWorld=Stored Integer
  MCU2_ControllerOverTemp_O : Constant  Value=0  OutDataTypeStr=single
  MCU2_ControllerOverTemp_S : ArithShift  BitShiftNumber=4
  MCU2_ControllerOverTemp_Sub : Subsystem
  MCU2_ControllerOverTemp_sat : Saturate  UpperLimit=3  LowerLimit=0
  MCU2_ControllerOverTempcv : DataTypeConversion
  MCU2_ControllerOverload_Ad : Sum
  MCU2_ControllerOverload_Convert : DataTypeConversion  OutDataTypeStr=uint32
  MCU2_ControllerOverload_F : Gain
  MCU2_ControllerOverload_L : simulink/Logic and Bit Operations/Bitwise Operator  logicop=AND  UseBitMask=on  BitMask=3  BitMaskRealWorld=Stored Integer
  MCU2_ControllerOverload_O : Constant  Value=0  OutDataTypeStr=single
  MCU2_ControllerOverload_S : ArithShift
  MCU2_ControllerOverload_Sub : Subsystem
  MCU2_ControllerOverload_sat : Saturate  UpperLimit=3  LowerLimit=0
  MCU2_ControllerOverloadcv : DataTypeConversion
  MCU2_DownratingFault_Ad : Sum
  MCU2_DownratingFault_Convert : DataTypeConversion  OutDataTypeStr=uint32
  MCU2_DownratingFault_F : Gain
  MCU2_DownratingFault_L : simulink/Logic and Bit Operations/Bitwise Operator  logicop=AND  UseBitMask=on  BitMask=192  BitMaskRealWorld=Stored Integer
  MCU2_DownratingFault_O : Constant  Value=0  OutDataTypeStr=single
  MCU2_DownratingFault_S : ArithShift  BitShiftNumber=6
  MCU2_DownratingFault_Sub : Subsystem
  MCU2_DownratingFault_sat : Saturate  UpperLimit=3  LowerLimit=0
  MCU2_DownratingFaultcv : DataTypeConversion
  MCU2_FaultLevel_Ad : Sum
  MCU2_FaultLevel_Convert : DataTypeConversion  OutDataTypeStr=uint32
  MCU2_FaultLevel_F : Gain
  MCU2_FaultLevel_L : simulink/Logic and Bit Operations/Bitwise Operator  logicop=AND  UseBitMask=on  BitMask=192  BitMaskRealWorld=Stored Integer
  MCU2_FaultLevel_O : Constant  Value=0  OutDataTypeStr=single
  MCU2_FaultLevel_S : ArithShift  BitShiftNumber=6
  MCU2_FaultLevel_Sub : Subsystem
  MCU2_FaultLevel_sat : Saturate  UpperLimit=3  LowerLimit=0
  MCU2_FaultLevelcv : DataTypeConversion
  MCU2_IGBTFault_Ad : Sum
  MCU2_IGBTFault_Convert : DataTypeConversion  OutDataTypeStr=uint32
  MCU2_IGBTFault_F : Gain
  MCU2_IGBTFault_L : simulink/Logic and Bit Operations/Bitwise Operator  logicop=AND  UseBitMask=on  BitMask=3  BitMaskRealWorld=Stored Integer
  MCU2_IGBTFault_O : Constant  Value=0  OutDataTypeStr=single
  MCU2_IGBTFault_S : ArithShift
  MCU2_IGBTFault_Sub : Subsystem
  MCU2_IGBTFault_sat : Saturate  UpperLimit=3  LowerLimit=0
  MCU2_IGBTFaultcv : DataTypeConversion
  MCU2_IdcSensorFault_Ad : Sum
  MCU2_IdcSensorFault_Convert : DataTypeConversion  OutDataTypeStr=uint32
  MCU2_IdcSensorFault_F : Gain
  MCU2_IdcSensorFault_L : simulink/Logic and Bit Operations/Bitwise Operator  logicop=AND  UseBitMask=on  BitMask=3  BitMaskRealWorld=Stored Integer
  MCU2_IdcSensorFault_O : Constant  Value=0  OutDataTypeStr=single
  MCU2_IdcSensorFault_S : ArithShift
  MCU2_IdcSensorFault_Sub : Subsystem
  MCU2_IdcSensorFault_sat : Saturate  UpperLimit=3  LowerLimit=0
  MCU2_IdcSensorFaultcv : DataTypeConversion
  MCU2_IuSensorFault_Ad : Sum
  MCU2_IuSensorFault_Convert : DataTypeConversion  OutDataTypeStr=uint32
  MCU2_IuSensorFault_F : Gain
  MCU2_IuSensorFault_L : simulink/Logic and Bit Operations/Bitwise Operator  logicop=AND  UseBitMask=on  BitMask=12  BitMaskRealWorld=Stored Integer
  MCU2_IuSensorFault_O : Constant  Value=0  OutDataTypeStr=single
  MCU2_IuSensorFault_S : ArithShift  BitShiftNumber=2
  MCU2_IuSensorFault_Sub : Subsystem
  MCU2_IuSensorFault_sat : Saturate  UpperLimit=3  LowerLimit=0
  MCU2_IuSensorFaultcv : DataTypeConversion
  MCU2_IvSensorFault_Ad : Sum
  MCU2_IvSensorFault_Convert : DataTypeConversion  OutDataTypeStr=uint32
  MCU2_IvSensorFault_F : Gain
  MCU2_IvSensorFault_L : simulink/Logic and Bit Operations/Bitwise Operator  logicop=AND  UseBitMask=on  BitMask=48  BitMaskRealWorld=Stored Integer
  MCU2_IvSensorFault_O : Constant  Value=0  OutDataTypeStr=single
  MCU2_IvSensorFault_S : ArithShift  BitShiftNumber=4
  MCU2_IvSensorFault_Sub : Subsystem
  MCU2_IvSensorFault_sat : Saturate  UpperLimit=3  LowerLimit=0
  MCU2_IvSensorFaultcv : DataTypeConversion
  MCU2_MemoryFault_Ad : Sum
  MCU2_MemoryFault_Convert : DataTypeConversion  OutDataTypeStr=uint32
  MCU2_MemoryFault_F : Gain
  MCU2_MemoryFault_L : simulink/Logic and Bit Operations/Bitwise Operator  logicop=AND  UseBitMask=on  BitMask=48  BitMaskRealWorld=Stored Integer
  MCU2_MemoryFault_O : Constant  Value=0  OutDataTypeStr=single
  MCU2_MemoryFault_S : ArithShift  BitShiftNumber=4
  MCU2_MemoryFault_Sub : Subsystem
  MCU2_MemoryFault_sat : Saturate  UpperLimit=3  LowerLimit=0
  MCU2_MemoryFaultcv : DataTypeConversion
  MCU2_MotorOverLoad_Ad : Sum
  MCU2_MotorOverLoad_Convert : DataTypeConversion  OutDataTypeStr=uint32
  MCU2_MotorOverLoad_F : Gain
  MCU2_MotorOverLoad_L : simulink/Logic and Bit Operations/Bitwise Operator  logicop=AND  UseBitMask=on  BitMask=3  BitMaskRealWorld=Stored Integer
  MCU2_MotorOverLoad_O : Constant  Value=0  OutDataTypeStr=single
  MCU2_MotorOverLoad_S : ArithShift
  MCU2_MotorOverLoad_Sub : Subsystem
  MCU2_MotorOverLoad_sat : Saturate  UpperLimit=3  LowerLimit=0
  MCU2_MotorOverLoadcv : DataTypeConversion
  MCU2_MotorOverSpeed_Ad : Sum
  MCU2_MotorOverSpeed_Convert : DataTypeConversion  OutDataTypeStr=uint32
  MCU2_MotorOverSpeed_F : Gain
  MCU2_MotorOverSpeed_L : simulink/Logic and Bit Operations/Bitwise Operator  logicop=AND  UseBitMask=on  BitMask=192  BitMaskRealWorld=Stored Integer
  MCU2_MotorOverSpeed_O : Constant  Value=0  OutDataTypeStr=single
  MCU2_MotorOverSpeed_S : ArithShift  BitShiftNumber=6
  MCU2_MotorOverSpeed_Sub : Subsystem
  MCU2_MotorOverSpeed_sat : Saturate  UpperLimit=3  LowerLimit=0
  MCU2_MotorOverSpeedcv : DataTypeConversion
  MCU2_MotorOverTemp_Ad : Sum
  MCU2_MotorOverTemp_Convert : DataTypeConversion  OutDataTypeStr=uint32
  MCU2_MotorOverTemp_F : Gain
  MCU2_MotorOverTemp_L : simulink/Logic and Bit Operations/Bitwise Operator  logicop=AND  UseBitMask=on  BitMask=12  BitMaskRealWorld=Stored Integer
  MCU2_MotorOverTemp_O : Constant  Value=0  OutDataTypeStr=single
  MCU2_MotorOverTemp_S : ArithShift  BitShiftNumber=2
  MCU2_MotorOverTemp_Sub : Subsystem
  MCU2_MotorOverTemp_sat : Saturate  UpperLimit=3  LowerLimit=0
  MCU2_MotorOverTempcv : DataTypeConversion
  MCU2_MotorStallingFault_Ad : Sum
  MCU2_MotorStallingFault_Convert : DataTypeConversion  OutDataTypeStr=uint32
  MCU2_MotorStallingFault_F : Gain
  MCU2_MotorStallingFault_L : simulink/Logic and Bit Operations/Bitwise Operator  logicop=AND  UseBitMask=on  BitMask=12  BitMaskRealWorld=Stored Integer
  MCU2_MotorStallingFault_O : Constant  Value=0  OutDataTypeStr=single
  MCU2_MotorStallingFault_S : ArithShift  BitShiftNumber=2
  MCU2_MotorStallingFault_Sub : Subsystem
  MCU2_MotorStallingFault_sat : Saturate  UpperLimit=3  LowerLimit=0
  MCU2_MotorStallingFaultcv : DataTypeConversion
  MCU2_OverVoltage_Ad : Sum
  MCU2_OverVoltage_Convert : DataTypeConversion  OutDataTypeStr=uint32
  MCU2_OverVoltage_F : Gain
  MCU2_OverVoltage_L : simulink/Logic and Bit Operations/Bitwise Operator  logicop=AND  UseBitMask=on  BitMask=12  BitMaskRealWorld=Stored Integer
  MCU2_OverVoltage_O : Constant  Value=0  OutDataTypeStr=single
  MCU2_OverVoltage_S : ArithShift  BitShiftNumber=2
  MCU2_OverVoltage_Sub : Subsystem
  MCU2_OverVoltage_sat : Saturate  UpperLimit=3  LowerLimit=0
  MCU2_OverVoltagecv : DataTypeConversion
  MCU2_RotaryInverterFault_Ad : Sum
  MCU2_RotaryInverterFault_Convert : DataTypeConversion  OutDataTypeStr=uint32
  MCU2_RotaryInverterFault_F : Gain
  MCU2_RotaryInverterFault_L : simulink/Logic and Bit Operations/Bitwise Operator  logicop=AND  UseBitMask=on  BitMask=192  BitMaskRealWorld=Stored Integer
  MCU2_RotaryInverterFault_O : Constant  Value=0  OutDataTypeStr=single
  MCU2_RotaryInverterFault_S : ArithShift  BitShiftNumber=6
  MCU2_RotaryInverterFault_Sub : Subsystem
  MCU2_RotaryInverterFault_sat : Saturate  UpperLimit=3  LowerLimit=0
  MCU2_RotaryInverterFaultcv : DataTypeConversion
  MCU2_TempSensorFault_Ad : Sum
  MCU2_TempSensorFault_Convert : DataTypeConversion  OutDataTypeStr=uint32
  MCU2_TempSensorFault_F : Gain
  MCU2_TempSensorFault_L : simulink/Logic and Bit Operations/Bitwise Operator  logicop=AND  UseBitMask=on  BitMask=3  BitMaskRealWorld=Stored Integer
  MCU2_TempSensorFault_O : Constant  Value=0  OutDataTypeStr=single
  MCU2_TempSensorFault_S : ArithShift
  MCU2_TempSensorFault_Sub : Subsystem
  MCU2_TempSensorFault_sat : Saturate  UpperLimit=3  LowerLimit=0
  MCU2_TempSensorFaultcv : DataTypeConversion
  MCU2_UdcDetectionFault_Ad : Sum
  MCU2_UdcDetectionFault_Convert : DataTypeConversion  OutDataTypeStr=uint32
  MCU2_UdcDetectionFault_F : Gain
  MCU2_UdcDetectionFault_L : simulink/Logic and Bit Operations/Bitwise Operator  logicop=AND  UseBitMask=on  BitMask=3  BitMaskRealWorld=Stored Integer
  MCU2_UdcDetectionFault_O : Constant  Value=0  OutDataTypeStr=single
  MCU2_UdcDetectionFault_S : ArithShift
  MCU2_UdcDetectionFault_Sub : Subsystem
  MCU2_UdcDetectionFault_sat : Saturate  UpperLimit=3  LowerLimit=0
  MCU2_UdcDetectionFaultcv : DataTypeConversion
  MCU2_UnderVoltage_Ad : Sum
  MCU2_UnderVoltage_Convert : DataTypeConversion  OutDataTypeStr=uint32
  MCU2_UnderVoltage_F : Gain
  MCU2_UnderVoltage_L : simulink/Logic and Bit Operations/Bitwise Operator  logicop=AND  UseBitMask=on  BitMask=48  BitMaskRealWorld=Stored Integer
  MCU2_UnderVoltage_O : Constant  Value=0  OutDataTypeStr=single
  MCU2_UnderVoltage_S : ArithShift  BitShiftNumber=4
  MCU2_UnderVoltage_Sub : Subsystem
  MCU2_UnderVoltage_sat : Saturate  UpperLimit=3  LowerLimit=0
  MCU2_UnderVoltagecv : DataTypeConversion
  MCU2_MotorStallingFault_Out : Outport
  MCU2_UdcDetectionFault_Out : Outport  Port=2
  MCU2_TempSensorFault_Out : Outport  Port=3
  MCU2_ActieDischargingFault_Out : Outport  Port=4
  MCU2_IdcSensorFault_Out : Outport  Port=5
  MCU2_IuSensorFault_Out : Outport  Port=6
  MCU2_IvSensorFault_Out : Outport  Port=7
  MCU2_FaultLevel_Out : Outport  Port=8
  MCU2_ControllerOverload_Out : Outport  Port=9
  MCU2_CanCommunicationFault_Out : Outport  Port=10
  MCU2_MemoryFault_Out : Outport  Port=11
  MCU2_DownratingFault_Out : Outport  Port=12
  MCU2_IGBTFault_Out : Outport  Port=13
  MCU2_MotorOverTemp_Out : Outport  Port=14
  MCU2_ControllerOverTemp_Out : Outport  Port=15
  MCU2_MotorOverSpeed_Out : Outport  Port=16
  MCU2_RotaryInverterFault_Out : Outport  Port=17
  MCU2_UnderVoltage_Out : Outport  Port=18
  MCU2_OverVoltage_Out : Outport  Port=19
  MCU2_MotorOverLoad_Out : Outport  Port=20
  wires:
  MCU2_MotorStallingFault_F/1 -> MCU2_MotorStallingFault_Ad/1
  MCU2_MotorStallingFault_O/1 -> MCU2_MotorStallingFault_Ad/2
  MCU2_MotorStallingFault_Ad/1 -> MCU2_MotorStallingFault_sat/1
  MCU2_MotorStallingFault_sat/1 -> MCU2_MotorStallingFault_Out/1
  Demux/6 -> MCU2_MotorStallingFault_Sub/1(In1), MCU2_UdcDetectionFault_Sub/1(In1)
  MCU2_MotorStallingFault_Sub/1(Out1) -> MCU2_MotorStallingFault_Convert/1
  MCU2_MotorStallingFault_Convert/1 -> MCU2_MotorStallingFault_L/1
  MCU2_MotorStallingFault_L/1 -> MCU2_MotorStallingFault_S/1
  MCU2_MotorStallingFault_S/1 -> MCU2_MotorStallingFaultcv/1
  MCU2_MotorStallingFaultcv/1 -> MCU2_MotorStallingFault_F/1
  MCU2_UdcDetectionFault_F/1 -> MCU2_UdcDetectionFault_Ad/1
  MCU2_UdcDetectionFault_O/1 -> MCU2_UdcDetectionFault_Ad/2
  MCU2_UdcDetectionFault_Ad/1 -> MCU2_UdcDetectionFault_sat/1
  MCU2_UdcDetectionFault_sat/1 -> MCU2_UdcDetectionFault_Out/1
  MCU2_UdcDetectionFault_Sub/1(Out1) -> MCU2_UdcDetectionFault_Convert/1
  MCU2_UdcDetectionFault_Convert/1 -> MCU2_UdcDetectionFault_L/1
  MCU2_UdcDetectionFault_L/1 -> MCU2_UdcDetectionFault_S/1
  MCU2_UdcDetectionFault_S/1 -> MCU2_UdcDetectionFaultcv/1
  MCU2_UdcDetectionFaultcv/1 -> MCU2_UdcDetectionFault_F/1
  MCU2_TempSensorFault_F/1 -> MCU2_TempSensorFault_Ad/1
  MCU2_TempSensorFault_O/1 -> MCU2_TempSensorFault_Ad/2
  MCU2_TempSensorFault_Ad/1 -> MCU2_TempSensorFault_sat/1
  MCU2_TempSensorFault_sat/1 -> MCU2_TempSensorFault_Out/1
  Demux/5 -> MCU2_TempSensorFault_Sub/1(In1), MCU2_ActieDischargingFault_Sub/1(In1)
  MCU2_TempSensorFault_Sub/1(Out1) -> MCU2_TempSensorFault_Convert/1
  MCU2_TempSensorFault_Convert/1 -> MCU2_TempSensorFault_L/1
  MCU2_TempSensorFault_L/1 -> MCU2_TempSensorFault_S/1
  MCU2_TempSensorFault_S/1 -> MCU2_TempSensorFaultcv/1
  MCU2_TempSensorFaultcv/1 -> MCU2_TempSensorFault_F/1
  MCU2_ActieDischargingFault_F/1 -> MCU2_ActieDischargingFault_Ad/1
  MCU2_ActieDischargingFault_O/1 -> MCU2_ActieDischargingFault_Ad/2
  MCU2_ActieDischargingFault_Ad/1 -> MCU2_ActieDischargingFault_sat/1
  MCU2_ActieDischargingFault_sat/1 -> MCU2_ActieDischargingFault_Out/1
  MCU2_ActieDischargingFault_Sub/1(Out1) -> MCU2_ActieDischargingFault_Convert/1
  MCU2_ActieDischargingFault_Convert/1 -> MCU2_ActieDischargingFault_L/1
  MCU2_ActieDischargingFault_L/1 -> MCU2_ActieDischargingFault_S/1
  MCU2_ActieDischargingFault_S/1 -> MCU2_ActieDischargingFaultcv/1
  MCU2_ActieDischargingFaultcv/1 -> MCU2_ActieDischargingFault_F/1
  MCU2_IdcSensorFault_F/1 -> MCU2_IdcSensorFault_Ad/1
  MCU2_IdcSensorFault_O/1 -> MCU2_IdcSensorFault_Ad/2
  MCU2_IdcSensorFault_Ad/1 -> MCU2_IdcSensorFault_sat/1
  MCU2_IdcSensorFault_sat/1 -> MCU2_IdcSensorFault_Out/1
  Demux/4 -> MCU2_IdcSensorFault_Sub/1(In1), MCU2_IuSensorFault_Sub/1(In1), MCU2_IvSensorFault_Sub/1(In1), MCU2_FaultLevel_Sub/1(In1)
  MCU2_IdcSensorFault_Sub/1(Out1) -> MCU2_IdcSensorFault_Convert/1
  MCU2_IdcSensorFault_Convert/1 -> MCU2_IdcSensorFault_L/1
  MCU2_IdcSensorFault_L/1 -> MCU2_IdcSensorFault_S/1
  MCU2_IdcSensorFault_S/1 -> MCU2_IdcSensorFaultcv/1
  MCU2_IdcSensorFaultcv/1 -> MCU2_IdcSensorFault_F/1
  MCU2_IuSensorFault_F/1 -> MCU2_IuSensorFault_Ad/1
  MCU2_IuSensorFault_O/1 -> MCU2_IuSensorFault_Ad/2
  MCU2_IuSensorFault_Ad/1 -> MCU2_IuSensorFault_sat/1
  MCU2_IuSensorFault_sat/1 -> MCU2_IuSensorFault_Out/1
  MCU2_IuSensorFault_Sub/1(Out1) -> MCU2_IuSensorFault_Convert/1
  MCU2_IuSensorFault_Convert/1 -> MCU2_IuSensorFault_L/1
  MCU2_IuSensorFault_L/1 -> MCU2_IuSensorFault_S/1
  MCU2_IuSensorFault_S/1 -> MCU2_IuSensorFaultcv/1
  MCU2_IuSensorFaultcv/1 -> MCU2_IuSensorFault_F/1
  MCU2_IvSensorFault_F/1 -> MCU2_IvSensorFault_Ad/1
  MCU2_IvSensorFault_O/1 -> MCU2_IvSensorFault_Ad/2
  MCU2_IvSensorFault_Ad/1 -> MCU2_IvSensorFault_sat/1
  MCU2_IvSensorFault_sat/1 -> MCU2_IvSensorFault_Out/1
  MCU2_IvSensorFault_Sub/1(Out1) -> MCU2_IvSensorFault_Convert/1
  MCU2_IvSensorFault_Convert/1 -> MCU2_IvSensorFault_L/1
  MCU2_IvSensorFault_L/1 -> MCU2_IvSensorFault_S/1
  MCU2_IvSensorFault_S/1 -> MCU2_IvSensorFaultcv/1
  MCU2_IvSensorFaultcv/1 -> MCU2_IvSensorFault_F/1
  MCU2_FaultLevel_F/1 -> MCU2_FaultLevel_Ad/1
  MCU2_FaultLevel_O/1 -> MCU2_FaultLevel_Ad/2
  MCU2_FaultLevel_Ad/1 -> MCU2_FaultLevel_sat/1
  MCU2_FaultLevel_sat/1 -> MCU2_FaultLevel_Out/1
  MCU2_FaultLevel_Sub/1(Out1) -> MCU2_FaultLevel_Convert/1
  MCU2_FaultLevel_Convert/1 -> MCU2_FaultLevel_L/1
  MCU2_FaultLevel_L/1 -> MCU2_FaultLevel_S/1
  MCU2_FaultLevel_S/1 -> MCU2_FaultLevelcv/1
  MCU2_FaultLevelcv/1 -> MCU2_FaultLevel_F/1
  MCU2_ControllerOverload_F/1 -> MCU2_ControllerOverload_Ad/1
  MCU2_ControllerOverload_O/1 -> MCU2_ControllerOverload_Ad/2
  MCU2_ControllerOverload_Ad/1 -> MCU2_ControllerOverload_sat/1
  MCU2_ControllerOverload_sat/1 -> MCU2_ControllerOverload_Out/1
  Demux/1 -> MCU2_UnderVoltage_Sub/1(In1), MCU2_OverVoltage_Sub/1(In1), MCU2_ControllerOverload_Sub/1(In1), MCU2_RotaryInverterFault_Sub/1(In1)
  MCU2_ControllerOverload_Sub/1(Out1) -> MCU2_ControllerOverload_Convert/1
  MCU2_ControllerOverload_Convert/1 -> MCU2_ControllerOverload_L/1
  MCU2_ControllerOverload_L/1 -> MCU2_ControllerOverload_S/1
  MCU2_ControllerOverload_S/1 -> MCU2_ControllerOverloadcv/1
  MCU2_ControllerOverloadcv/1 -> MCU2_ControllerOverload_F/1
  MCU2_CanCommunicationFault_F/1 -> MCU2_CanCommunicationFault_Ad/1
  MCU2_CanCommunicationFault_O/1 -> MCU2_CanCommunicationFault_Ad/2
  MCU2_CanCommunicationFault_Ad/1 -> MCU2_CanCommunicationFault_sat/1
  MCU2_CanCommunicationFault_sat/1 -> MCU2_CanCommunicationFault_Out/1
  Demux/3 -> MCU2_DownratingFault_Sub/1(In1), MCU2_MotorOverLoad_Sub/1(In1), MCU2_MemoryFault_Sub/1(In1), MCU2_CanCommunicationFault_Sub/1(In1)
  MCU2_CanCommunicationFault_Sub/1(Out1) -> MCU2_CanCommunicationFault_Convert/1
  MCU2_CanCommunicationFault_Convert/1 -> MCU2_CanCommunicationFault_L/1
  MCU2_CanCommunicationFault_L/1 -> MCU2_CanCommunicationFault_S/1
  MCU2_CanCommunicationFault_S/1 -> MCU2_CanCommunicationFaultcv/1
  MCU2_CanCommunicationFaultcv/1 -> MCU2_CanCommunicationFault_F/1
  MCU2_MemoryFault_F/1 -> MCU2_MemoryFault_Ad/1
  MCU2_MemoryFault_O/1 -> MCU2_MemoryFault_Ad/2
  MCU2_MemoryFault_Ad/1 -> MCU2_MemoryFault_sat/1
  MCU2_MemoryFault_sat/1 -> MCU2_MemoryFault_Out/1
  MCU2_MemoryFault_Sub/1(Out1) -> MCU2_MemoryFault_Convert/1
  MCU2_MemoryFault_Convert/1 -> MCU2_MemoryFault_L/1
  MCU2_MemoryFault_L/1 -> MCU2_MemoryFault_S/1
  MCU2_MemoryFault_S/1 -> MCU2_MemoryFaultcv/1
  MCU2_MemoryFaultcv/1 -> MCU2_MemoryFault_F/1
  MCU2_DownratingFault_F/1 -> MCU2_DownratingFault_Ad/1
  MCU2_DownratingFault_O/1 -> MCU2_DownratingFault_Ad/2
  MCU2_DownratingFault_Ad/1 -> MCU2_DownratingFault_sat/1
  MCU2_DownratingFault_sat/1 -> MCU2_DownratingFault_Out/1
  MCU2_DownratingFault_Sub/1(Out1) -> MCU2_DownratingFault_Convert/1
  MCU2_DownratingFault_Convert/1 -> MCU2_DownratingFault_L/1
  MCU2_DownratingFault_L/1 -> MCU2_DownratingFault_S/1
  MCU2_DownratingFault_S/1 -> MCU2_DownratingFaultcv/1
  MCU2_DownratingFaultcv/1 -> MCU2_DownratingFault_F/1
  MCU2_IGBTFault_F/1 -> MCU2_IGBTFault_Ad/1
  MCU2_IGBTFault_O/1 -> MCU2_IGBTFault_Ad/2
  MCU2_IGBTFault_Ad/1 -> MCU2_IGBTFault_sat/1
  MCU2_IGBTFault_sat/1 -> MCU2_IGBTFault_Out/1
  Demux/2 -> MCU2_ControllerOverTemp_Sub/1(In1), MCU2_MotorOverSpeed_Sub/1(In1), MCU2_IGBTFault_Sub/1(In1), MCU2_MotorOverTemp_Sub/1(In1)
  MCU2_IGBTFault_Sub/1(Out1) -> MCU2_IGBTFault_Convert/1
  MCU2_IGBTFault_Convert/1 -> MCU2_IGBTFault_L/1
  MCU2_IGBTFault_L/1 -> MCU2_IGBTFault_S/1
  MCU2_IGBTFault_S/1 -> MCU2_IGBTFaultcv/1
  MCU2_IGBTFaultcv/1 -> MCU2_IGBTFault_F/1
  MCU2_MotorOverTemp_F/1 -> MCU2_MotorOverTemp_Ad/1
  MCU2_MotorOverTemp_O/1 -> MCU2_MotorOverTemp_Ad/2
  MCU2_MotorOverTemp_Ad/1 -> MCU2_MotorOverTemp_sat/1
  MCU2_MotorOverTemp_sat/1 -> MCU2_MotorOverTemp_Out/1
  MCU2_MotorOverTemp_Sub/1(Out1) -> MCU2_MotorOverTemp_Convert/1
  MCU2_MotorOverTemp_Convert/1 -> MCU2_MotorOverTemp_L/1
  MCU2_MotorOverTemp_L/1 -> MCU2_MotorOverTemp_S/1
  MCU2_MotorOverTemp_S/1 -> MCU2_MotorOverTempcv/1
  MCU2_MotorOverTempcv/1 -> MCU2_MotorOverTemp_F/1
  MCU2_ControllerOverTemp_F/1 -> MCU2_ControllerOverTemp_Ad/1
  MCU2_ControllerOverTemp_O/1 -> MCU2_ControllerOverTemp_Ad/2
  MCU2_ControllerOverTemp_Ad/1 -> MCU2_ControllerOverTemp_sat/1
  MCU2_ControllerOverTemp_sat/1 -> MCU2_ControllerOverTemp_Out/1
  MCU2_ControllerOverTemp_Sub/1(Out1) -> MCU2_ControllerOverTemp_Convert/1
  MCU2_ControllerOverTemp_Convert/1 -> MCU2_ControllerOverTemp_L/1
  MCU2_ControllerOverTemp_L/1 -> MCU2_ControllerOverTemp_S/1
  MCU2_ControllerOverTemp_S/1 -> MCU2_ControllerOverTempcv/1
  MCU2_ControllerOverTempcv/1 -> MCU2_ControllerOverTemp_F/1
  MCU2_MotorOverSpeed_F/1 -> MCU2_MotorOverSpeed_Ad/1
  MCU2_MotorOverSpeed_O/1 -> MCU2_MotorOverSpeed_Ad/2
  MCU2_MotorOverSpeed_Ad/1 -> MCU2_MotorOverSpeed_sat/1
  MCU2_MotorOverSpeed_sat/1 -> MCU2_MotorOverSpeed_Out/1
  MCU2_MotorOverSpeed_Sub/1(Out1) -> MCU2_MotorOverSpeed_Convert/1
  MCU2_MotorOverSpeed_Convert/1 -> MCU2_MotorOverSpeed_L/1
  MCU2_MotorOverSpeed_L/1 -> MCU2_MotorOverSpeed_S/1
  MCU2_MotorOverSpeed_S/1 -> MCU2_MotorOverSpeedcv/1
  MCU2_MotorOverSpeedcv/1 -> MCU2_MotorOverSpeed_F/1
  MCU2_RotaryInverterFault_F/1 -> MCU2_RotaryInverterFault_Ad/1
  MCU2_RotaryInverterFault_O/1 -> MCU2_RotaryInverterFault_Ad/2
  MCU2_RotaryInverterFault_Ad/1 -> MCU2_RotaryInverterFault_sat/1
  MCU2_RotaryInverterFault_sat/1 -> MCU2_RotaryInverterFault_Out/1
  MCU2_RotaryInverterFault_Sub/1(Out1) -> MCU2_RotaryInverterFault_Convert/1
  MCU2_RotaryInverterFault_Convert/1 -> MCU2_RotaryInverterFault_L/1
  MCU2_RotaryInverterFault_L/1 -> MCU2_RotaryInverterFault_S/1
  MCU2_RotaryInverterFault_S/1 -> MCU2_RotaryInverterFaultcv/1
  MCU2_RotaryInverterFaultcv/1 -> MCU2_RotaryInverterFault_F/1
  MCU2_UnderVoltage_F/1 -> MCU2_UnderVoltage_Ad/1
  MCU2_UnderVoltage_O/1 -> MCU2_UnderVoltage_Ad/2
  MCU2_UnderVoltage_Ad/1 -> MCU2_UnderVoltage_sat/1
  MCU2_UnderVoltage_sat/1 -> MCU2_UnderVoltage_Out/1
  MCU2_UnderVoltage_Sub/1(Out1) -> MCU2_UnderVoltage_Convert/1
  MCU2_UnderVoltage_Convert/1 -> MCU2_UnderVoltage_L/1
  MCU2_UnderVoltage_L/1 -> MCU2_UnderVoltage_S/1
  MCU2_UnderVoltage_S/1 -> MCU2_UnderVoltagecv/1
  MCU2_UnderVoltagecv/1 -> MCU2_UnderVoltage_F/1
  MCU2_OverVoltage_F/1 -> MCU2_OverVoltage_Ad/1
  MCU2_OverVoltage_O/1 -> MCU2_OverVoltage_Ad/2
  MCU2_OverVoltage_Ad/1 -> MCU2_OverVoltage_sat/1
  MCU2_OverVoltage_sat/1 -> MCU2_OverVoltage_Out/1
  MCU2_OverVoltage_Sub/1(Out1) -> MCU2_OverVoltage_Convert/1
  MCU2_OverVoltage_Convert/1 -> MCU2_OverVoltage_L/1
  MCU2_OverVoltage_L/1 -> MCU2_OverVoltage_S/1
  MCU2_OverVoltage_S/1 -> MCU2_OverVoltagecv/1
  MCU2_OverVoltagecv/1 -> MCU2_OverVoltage_F/1
  MCU2_MotorOverLoad_F/1 -> MCU2_MotorOverLoad_Ad/1
  MCU2_MotorOverLoad_O/1 -> MCU2_MotorOverLoad_Ad/2
  MCU2_MotorOverLoad_Ad/1 -> MCU2_MotorOverLoad_sat/1
  MCU2_MotorOverLoad_sat/1 -> MCU2_MotorOverLoad_Out/1
  MCU2_MotorOverLoad_Sub/1(Out1) -> MCU2_MotorOverLoad_Convert/1
  MCU2_MotorOverLoad_Convert/1 -> MCU2_MotorOverLoad_L/1
  MCU2_MotorOverLoad_L/1 -> MCU2_MotorOverLoad_S/1
  MCU2_MotorOverLoad_S/1 -> MCU2_MotorOverLoadcv/1
  MCU2_MotorOverLoadcv/1 -> MCU2_MotorOverLoad_F/1
  input/1 -> Demux/1

== matlab function six_plus_six_AcmsteeringV10_main/MainControl/mode_control/forward/forward/Drive/驱动防滑控制TCS/直行TCS/直行/MATLAB Function ==
  data: s_act_lf input; flag_lf output; s_opt_zhuan input; s_opt_zhuan_add input; flag_lf_pre input int8
function flag_lf = fcn(s_act_lf,s_opt_zhuan,s_opt_zhuan_add,flag_lf_pre)
%#codegen
if s_act_lf>s_opt_zhuan+s_opt_zhuan_add
    flag_lf=int8(1);
elseif s_act_lf<s_opt_zhuan
    flag_lf =int8(0);
else
    flag_lf=int8(flag_lf_pre);
end
end
